simulink model "case2"  (R2024a)
settings: Solver=VariableStepAuto  StartTime=0.0  StopTime=10.0  RelTol=1e-3
settings Model: Creator=tusha  LastModifiedBy=tusha

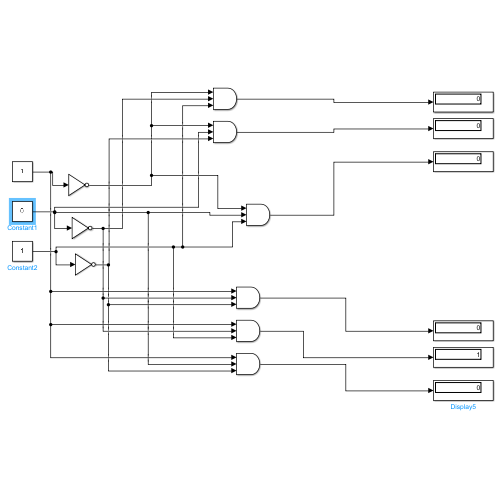
[thumbnail: Simulink's stored preview of the top-level diagram]
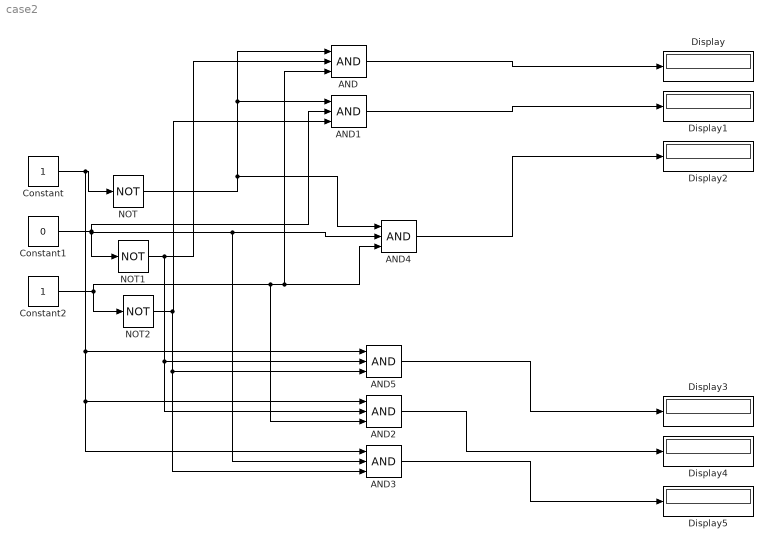
== system case2 ==
  AND{,1..5} (6 alike) : Logic  Inputs=3  IconShape=distinctive  AllPortsSameDT=off  OutDataTypeStr=boolean
  Constant : Constant
  Constant1 : Constant  Value=0
  Constant2 : Constant
  Display{,1..5} (6 alike) : Display
  NOT : Logic  Operator=NOT  IconShape=distinctive  AllPortsSameDT=off  OutDataTypeStr=boolean
  NOT1 : Logic  Operator=NOT  IconShape=distinctive  AllPortsSameDT=off  OutDataTypeStr=boolean
  NOT2 : Logic  Operator=NOT  IconShape=distinctive  AllPortsSameDT=off  OutDataTypeStr=boolean
  wires:
  Constant/1 -> AND3/1, AND2/1, AND5/1, NOT/1
  Constant1/1 -> NOT1/1, AND3/2, AND4/2, AND1/2
  Constant2/1 -> AND2/3, AND4/3, AND/3, NOT2/1
  NOT/1 -> AND1/1, AND/1, AND4/1
  NOT1/1 -> AND2/2, AND5/2, AND/2
  AND/1 -> Display/1
  AND1/1 -> Display1/1
  AND4/1 -> Display2/1
  AND5/1 -> Display3/1
  AND2/1 -> Display4/1
  AND3/1 -> Display5/1
  NOT2/1 -> AND3/3, AND5/3, AND1/3
